simulink model "CF018A_GmRoadWhlInQlfr"  (R2013b)
settings: Solver=FixedStepDiscrete  SolverMode=SingleTasking  StartTime=0.0  StopTime=1  FixedStep=0.002  RelTol=1e-3
values from neighbouring files (symbols this model uses):
  DELTAPLSROLLOVR_CNT_S16 = DataDict.Constant    [CF018A_GmRoadWhlInQlfr_DataDict.m]
  DELTATISTAMPCNTROLLOVR_CNT_S32 = DataDict.Constant    [CF018A_GmRoadWhlInQlfr_DataDict.m]
  GmRoadWhlInQlfrMaxAllwblFrq = DataDict.Calibration    [CF018A_GmRoadWhlInQlfr_DataDict.m]
  GmRoadWhlInQlfrMaxFrqChg = DataDict.Calibration    [CF018A_GmRoadWhlInQlfr_DataDict.m]
  LEFRQCHGOUTOFRNG_CNT_U08 = DataDict.Constant    [CF018A_GmRoadWhlInQlfr_DataDict.m]
  LEFRQOUTOFRNG_CNT_U08 = DataDict.Constant    [CF018A_GmRoadWhlInQlfr_DataDict.m]
  NODEBSTEP_CNT_U16 = DataDict.Constant    [CF018A_GmRoadWhlInQlfr_DataDict.m]
  PARKDURN_CNT_F32 = DataDict.Constant    [CF018A_GmRoadWhlInQlfr_DataDict.m]
  PREVRAWWHLFRQMIN_HZ_F32 = DataDict.Constant    [CF018A_GmRoadWhlInQlfr_DataDict.m]
  RIFRQCHGOUTOFRNG_CNT_U08 = DataDict.Constant    [CF018A_GmRoadWhlInQlfr_DataDict.m]
  RIFRQOUTOFRNG_CNT_U08 = DataDict.Constant    [CF018A_GmRoadWhlInQlfr_DataDict.m]
  RoadWhlFrqInCalcOutOfRng = DataDict.NTC    [CF018A_GmRoadWhlInQlfr_DataDict.m]
  SECTO100MICROSECCNVN_CNT_F32 = DataDict.Constant    [CF018A_GmRoadWhlInQlfr_DataDict.m]
  WHLFRQMIN_HZ_F32 = DataDict.Constant    [CF018A_GmRoadWhlInQlfr_DataDict.m]
undefined symbols (not defined in the file or in its folder): NtcSts1
libraries: simulink x5, NxtrAbslt x2, NxtrLim x2
(part 3 of 5)

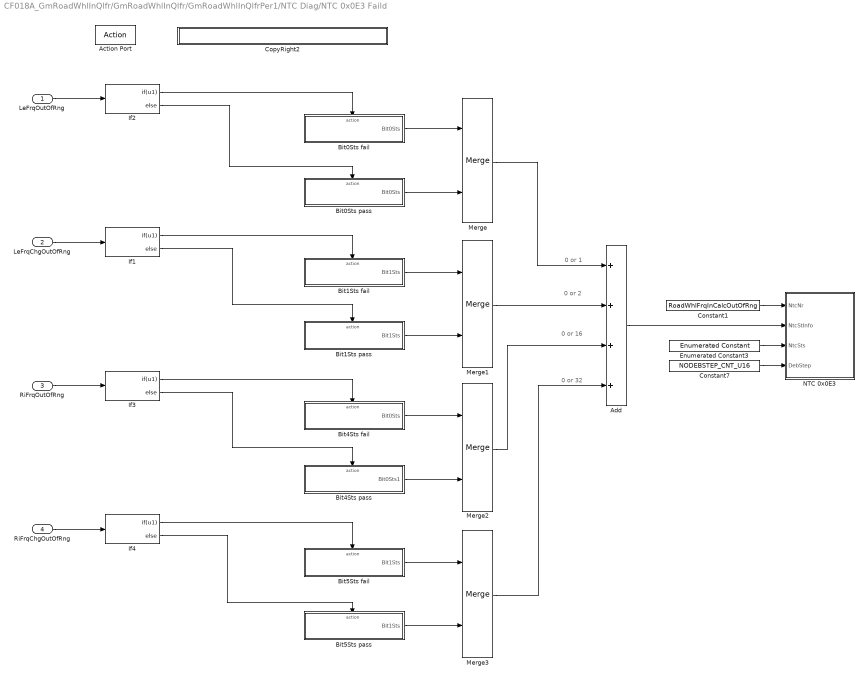
== system CF018A_GmRoadWhlInQlfr/GmRoadWhlInQlfr/GmRoadWhlInQlfrPer1/NTC Diag/NTC 0x0E3 Faild ==
  note: 0 or 32
  note: 0 or 16
  note: 0 or 2
  note: 0 or 1
  LeFrqOutOfRng : Inport  RequirementInfo="{'linktype_rmi_doors' '0000c6e7 (/GM T1XX/SubSystem Specifications/Customer Functions/CF018A GM Road Wheel Input Qualifier)' '#217' 'true' 'REQ:  217' '' } %GIDa_195ab2bc_dfff_4d6d_a0a2_4361903f55fa"
  LeFrqChgOutOfRng : Inport  RequirementInfo="{'linktype_rmi_doors' '0000c6e7 (/GM T1XX/SubSystem Specifications/Customer Functions/CF018A GM Road Wheel Input Qualifier)' '#219' 'true' 'REQ:  219' '' } %GIDa_52460b67_ef53_458f_9626_54e9bbcdf812"  Port=2
  RiFrqOutOfRng : Inport  RequirementInfo="{'linktype_rmi_doors' '0000c6e7 (/GM T1XX/SubSystem Specifications/Customer Functions/CF018A GM Road Wheel Input Qualifier)' '#220' 'true' 'REQ:  220' '' } %GIDa_71d41fd8_1e3e_427a_97ad_955d8ac34ef3"  Port=3
  RiFrqChgOutOfRng : Inport  RequirementInfo="{'linktype_rmi_doors' '0000c6e7 (/GM T1XX/SubSystem Specifications/Customer Functions/CF018A GM Road Wheel Input Qualifier)' '#221' 'true' 'REQ:  221' '' } %GIDa_232d1f07_579d_47ef_90f3_e50f36280ea6"  Port=4
  Action Port : ActionPort  ActionType=then
  Add : Sum  Inputs=++++
  Bit0Sts fail : Subsystem  RequirementInfo="{'linktype_rmi_doors' '0000c6e7 (/GM T1XX/SubSystem Specifications/Customer Functions/CF018A GM Road Wheel Input Qualifier)' '#217' 'true' 'REQ:  217' '' } %GIDa_14e418d7_b229_4493_b7eb_676a8f1cb482"  TreatAsAtomicUnit=on
  Bit0Sts pass : Subsystem  RequirementInfo="{'linktype_rmi_doors' '0000c6e7 (/GM T1XX/SubSystem Specifications/Customer Functions/CF018A GM Road Wheel Input Qualifier)' '#217' 'true' 'REQ:  217' '' } %GIDa_4b309baa_eb20_4fda_8a66_476882cf3a3c"  TreatAsAtomicUnit=on
  Bit1Sts fail : Subsystem  RequirementInfo="{'linktype_rmi_doors' '0000c6e7 (/GM T1XX/SubSystem Specifications/Customer Functions/CF018A GM Road Wheel Input Qualifier)' '#219' 'true' 'REQ:  219' '' } %GIDa_385de269_cf1d_4f17_ae75_b6c4c0e42b90"  TreatAsAtomicUnit=on
  Bit1Sts pass : Subsystem  RequirementInfo="{'linktype_rmi_doors' '0000c6e7 (/GM T1XX/SubSystem Specifications/Customer Functions/CF018A GM Road Wheel Input Qualifier)' '#219' 'true' 'REQ:  219' '' } %GIDa_8ec329c6_93d5_43d4_8a4f_e98046b859d6"  TreatAsAtomicUnit=on
  Bit4Sts fail : Subsystem  RequirementInfo="{'linktype_rmi_doors' '0000c6e7 (/GM T1XX/SubSystem Specifications/Customer Functions/CF018A GM Road Wheel Input Qualifier)' '#220' 'true' 'REQ:  220' '' } %GIDa_b3b904ac_bc0c_48f5_a89a_5cd3c3707194"  TreatAsAtomicUnit=on
  Bit4Sts pass : Subsystem  RequirementInfo="{'linktype_rmi_doors' '0000c6e7 (/GM T1XX/SubSystem Specifications/Customer Functions/CF018A GM Road Wheel Input Qualifier)' '#220' 'true' 'REQ:  220' '' } %GIDa_da90ecd1_a52b_401f_93fe_b339ee453102"  TreatAsAtomicUnit=on
  Bit5Sts fail : Subsystem  RequirementInfo="{'linktype_rmi_doors' '0000c6e7 (/GM T1XX/SubSystem Specifications/Customer Functions/CF018A GM Road Wheel Input Qualifier)' '#221' 'true' 'REQ:  221' '' } %GIDa_36f13dc0_335a_4247_a7fa_e2ce04f25d73"  TreatAsAtomicUnit=on
  Bit5Sts pass : Subsystem  RequirementInfo="{'linktype_rmi_doors' '0000c6e7 (/GM T1XX/SubSystem Specifications/Customer Functions/CF018A GM Road Wheel Input Qualifier)' '#221' 'true' 'REQ:  221' '' } %GIDa_8dbc0c8d_e7dc_445e_adc9_a51dc08e9455"  TreatAsAtomicUnit=on
  Constant1 : Constant  Value=RoadWhlFrqInCalcOutOfRng
  Constant7 : Constant  Value=NODEBSTEP_CNT_U16
  CopyRight2 : Subsystem  Description=|  mask(Copyright Information){none=on}
      | Copyright info block.                                               
      |                                                                     
      | Place copyright information at the top of every subsystem in design.
      mask prompts: none "No parameters"
      mask help: Place copyright information at the top of every subsystem in design.
      mask Display:
      | NxtrConf = 'Nexteer Confidential';
      | 
      | sys = bdroot; %handle for the current model ("system")
      | first = get_param(sys,'Created');
      | if(isempty(first))
      |     first = datestr(now,'yyyy');
      | else
      |     first = first(end-3:end);  %year is last four digits
      | end
      | 
      | last = get_param(sys,'LastModifiedDate');
      | if isempty(last)
      |     last = datestr(now,'yyyy');
      | else
      |     last = last(end-3:end);
      | end
      | 
      | if strcmp(first,last)
      |     fprintf('%s -- Copyright %s Nexteer',NxtrConf,first)
      | else
      |     fprintf('%s -- %s%s- %s Nexteer',NxtrConf,char(169),first,last)
      | end
  Enumerated Constant3 : simulink/Sources/Enumerated Constant  OutDataTypeStr=Enum: NtcSts1  Value=NtcSts1.NTCSTS_FAILD  SampleTime=inf
  If1 : If  RequirementInfo="{'linktype_rmi_doors' '0000c6e7 (/GM T1XX/SubSystem Specifications/Customer Functions/CF018A GM Road Wheel Input Qualifier)' '#219' 'true' 'REQ:  219' '' } %GIDa_aff6807a_1779_44a1_bb5d_bde3c1762c20"  IfExpression=u1
  If2 : If  RequirementInfo="{'linktype_rmi_doors' '0000c6e7 (/GM T1XX/SubSystem Specifications/Customer Functions/CF018A GM Road Wheel Input Qualifier)' '#217' 'true' 'REQ:  217' '' } %GIDa_a1263e25_a3bc_4e7a_be4f_bbb224f699c2"  IfExpression=u1
  If3 : If  RequirementInfo="{'linktype_rmi_doors' '0000c6e7 (/GM T1XX/SubSystem Specifications/Customer Functions/CF018A GM Road Wheel Input Qualifier)' '#220' 'true' 'REQ:  220' '' } %GIDa_0718b7b5_3f2c_43be_9873_dfe0614914d9"  IfExpression=u1
  If4 : If  RequirementInfo="{'linktype_rmi_doors' '0000c6e7 (/GM T1XX/SubSystem Specifications/Customer Functions/CF018A GM Road Wheel Input Qualifier)' '#221' 'true' 'REQ:  221' '' } %GIDa_596e93e5_c856_4c8d_b061_564bb26e16d1"  IfExpression=u1
  Merge : Merge  RequirementInfo="{'linktype_rmi_doors' '0000c6e7 (/GM T1XX/SubSystem Specifications/Customer Functions/CF018A GM Road Wheel Input Qualifier)' '#217' 'true' 'REQ:  217' '' } %GIDa_ff64cedf_763d_4ec6_811f_3d7fe7e08dc9"
  Merge1 : Merge  RequirementInfo="{'linktype_rmi_doors' '0000c6e7 (/GM T1XX/SubSystem Specifications/Customer Functions/CF018A GM Road Wheel Input Qualifier)' '#219' 'true' 'REQ:  219' '' } %GIDa_d687efa6_6282_443c_95ea_f8a69d949498"
  Merge2 : Merge  RequirementInfo="{'linktype_rmi_doors' '0000c6e7 (/GM T1XX/SubSystem Specifications/Customer Functions/CF018A GM Road Wheel Input Qualifier)' '#220' 'true' 'REQ:  220' '' } %GIDa_a420e449_a616_43ba_b126_66db9afefef1"
  Merge3 : Merge  RequirementInfo="{'linktype_rmi_doors' '0000c6e7 (/GM T1XX/SubSystem Specifications/Customer Functions/CF018A GM Road Wheel Input Qualifier)' '#221' 'true' 'REQ:  221' '' } %GIDa_6aea80f1_e3e4_4567_b723_2621865e42b7"
  NTC 0x0E3 : Subsystem  mask(SetNTC){}
      mask help: SetNTC library block
  wires:
  LeFrqOutOfRng/1 -> If2/1
  LeFrqChgOutOfRng/1 -> If1/1
  RiFrqOutOfRng/1 -> If3/1
  RiFrqChgOutOfRng/1 -> If4/1
  If2/1 -> Bit0Sts fail/Action
  If2/2 -> Bit0Sts pass/Action
  If1/1 -> Bit1Sts fail/Action
  If1/2 -> Bit1Sts pass/Action
  If3/1 -> Bit4Sts fail/Action
  If3/2 -> Bit4Sts pass/Action
  If4/1 -> Bit5Sts fail/Action
  If4/2 -> Bit5Sts pass/Action
  Bit0Sts fail/1(Bit0Sts) -> Merge/1
  Bit0Sts pass/1(Bit0Sts) -> Merge/2
  Bit1Sts fail/1(Bit1Sts) -> Merge1/1
  Bit1Sts pass/1(Bit1Sts) -> Merge1/2
  Bit4Sts fail/1(Bit0Sts) -> Merge2/1
  Bit4Sts pass/1(Bit0Sts1) -> Merge2/2
  Bit5Sts fail/1(Bit1Sts) -> Merge3/1
  Bit5Sts pass/1(Bit1Sts) -> Merge3/2
  Merge/1 -> Add/1
  Merge1/1 -> Add/2
  Merge2/1 -> Add/3
  Merge3/1 -> Add/4
  Enumerated Constant3/1 -> NTC 0x0E3/3(NtcSts)
  Constant7/1 -> NTC 0x0E3/4(DebStep)
  Add/1 -> NTC 0x0E3/2(NtcStInfo)
  Constant1/1 -> NTC 0x0E3/1(NtcNr)

== system CF018A_GmRoadWhlInQlfr/GmRoadWhlInQlfr/GmRoadWhlInQlfrPer1/NTC Diag/NTC 0x0E3 Passd ==
  NtcNr : Inport
  NtcStInfo : Inport  Port=2
  NtcSts : Inport  Port=3
  DebStep : Inport  Port=4
  CallDiagMgr : ActionPort  ActionType=else
  SetNtcSts : Subsystem  RequirementInfo={} %GIDa_11b0bea6_d358_4d89_9e51_342e19f776d7  TreatAsAtomicUnit=on
      settings: RTWSystemCode=Inline
  wires:
  NtcStInfo/1 -> SetNtcSts/2(NtcStInfo)
  DebStep/1 -> SetNtcSts/4(DebStep)
  NtcSts/1 -> SetNtcSts/3(NtcSts)
  NtcNr/1 -> SetNtcSts/1(NtcNr)  "NtcNr"

== system CF018A_GmRoadWhlInQlfr/GmRoadWhlInQlfr/GmRoadWhlInQlfrPer1/Set Min Le whl Frq and false /CopyRight2 ==

== system CF018A_GmRoadWhlInQlfr/GmRoadWhlInQlfr/GmRoadWhlInQlfrPer1/Set Min Ri whl Frq and false /CopyRight2 ==

== system CF018A_GmRoadWhlInQlfr/GmRoadWhlInQlfr/GmRoadWhlInQlfrInit1/NTC 0x0E3 Passd/SetNtcSts/CopyRight2 ==

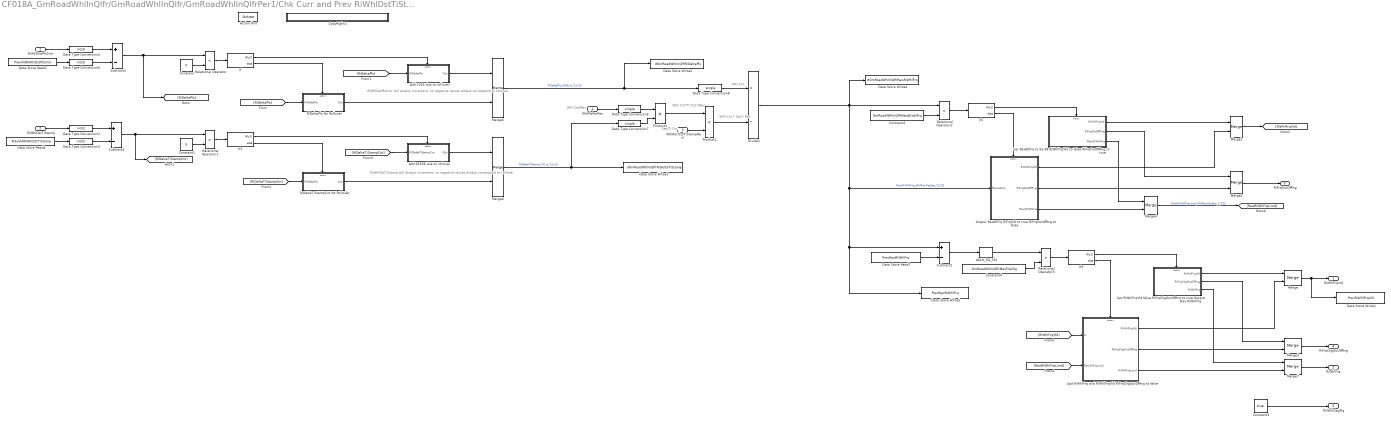
== system CF018A_GmRoadWhlInQlfr/GmRoadWhlInQlfr/GmRoadWhlInQlfrPer1/Chk Curr and Prev RiWhlDstTiStamp/Calc RiWhlFrq and RiWhlFrqVld /Calc RiWhlFrq and RiWhlFrqVld  ==
  note: RiWhlDstPlsCntr will always increment, so negative values always correspond to rollover
  note: RiWhlDstTiStamp will always increment, so negative values always correspond to rollover
  note: Whl Cnt/Rev
  note: Whl Cnt
  note: (Whl Cnt * Sec)/ Rev
  note: (Whl Cnt*Ti Cnt)/Rev
  note: Sec/Ti Cnt
  RiWhlDstPlsCntr : Inport  RequirementInfo="{'linktype_rmi_doors' '0000c6e7 (/GM T1XX/SubSystem Specifications/Customer Functions/CF018A GM Road Wheel Input Qualifier)' '#193' 'true' 'REQ:  193' '' } %GIDa_3e8ab2e0_17e6_46c6_9b5a_a415c584676f"
  RiWhlDstTiStamp : Inport  RequirementInfo="{'linktype_rmi_doors' '0000c6e7 (/GM T1XX/SubSystem Specifications/Customer Functions/CF018A GM Road Wheel Input Qualifier)' '#193' 'true' 'REQ:  193' '' } %GIDa_5cc4ad43_c4fb_48e7_9d1a_97e50fd9bb1d"  Port=2
  WhlRotlStsTiStampResl : Inport  RequirementInfo="{'linktype_rmi_doors' '0000c6e7 (/GM T1XX/SubSystem Specifications/Customer Functions/CF018A GM Road Wheel Input Qualifier)' '#193' 'true' 'REQ:  193' '' } %GIDa_18c1bb4c_4f3d_4131_89e1_1f0c775e5c47"  Port=3
  WhlPlsPerRev : Inport  RequirementInfo="{'linktype_rmi_doors' '0000c6e7 (/GM T1XX/SubSystem Specifications/Customer Functions/CF018A GM Road Wheel Input Qualifier)' '#193' 'true' 'REQ:  193' '' } %GIDa_22c598b2_0977_47f8_84d1_6d93f9add662"  Port=4
  Action Port : ActionPort  ActionType=then
  Abslt_f32_f32 : NxtrAbslt/Abslt_f32_f32  RequirementInfo="{'linktype_rmi_doors' '0000c6e7 (/GM T1XX/SubSystem Specifications/Customer Functions/CF018A GM Road Wheel Input Qualifier)' '#195' 'true' 'REQ:  195' '' } %GIDa_b87ef623_fea8_40fc_be2f_01a19a2481d3"  SFunctionSpec=single y1 = Abslt_f32_f32(single u1)
      settings: AttributesFormatString=%<Name>
  Add 1024 due to rollover : Subsystem  RequirementInfo="{'linktype_rmi_doors' '0000c6e7 (/GM T1XX/SubSystem Specifications/Customer Functions/CF018A GM Road Wheel Input Qualifier)' '#193' 'true' 'REQ:  193' '' } %GIDa_bbe013d7_37c0_4606_a70f_3e626e7cf5b9"  TreatAsAtomicUnit=on
  Add 65536 due to rollover : Subsystem  RequirementInfo="{'linktype_rmi_doors' '0000c6e7 (/GM T1XX/SubSystem Specifications/Customer Functions/CF018A GM Road Wheel Input Qualifier)' '#193' 'true' 'REQ:  193' '' } %GIDa_8f11591a_3e36_4330_89d4_3e165bb1c8e4"  TreatAsAtomicUnit=on
  Constant : Constant  RequirementInfo="{'linktype_rmi_doors' '0000c6e7 (/GM T1XX/SubSystem Specifications/Customer Functions/CF018A GM Road Wheel Input Qualifier)' '#193' 'true' 'REQ:  193' '' } %GIDa_b5ba1cba_4aae_479b_830a_1e93dfe9f490"  Value=0  OutDataTypeStr=int16
  Constant1 : Constant  RequirementInfo="{'linktype_rmi_doors' '0000c6e7 (/GM T1XX/SubSystem Specifications/Customer Functions/CF018A GM Road Wheel Input Qualifier)' '#193' 'true' 'REQ:  193' '' } %GIDa_e84f4047_7d95_4eef_aeae_45f6caa05096"  Value=0
  Constant2 : Constant  RequirementInfo="{'linktype_rmi_doors' '0000c6e7 (/GM T1XX/SubSystem Specifications/Customer Functions/CF018A GM Road Wheel Input Qualifier)' '#218' 'true' 'REQ:  218' '' ; 'linktype_rmi_doors' '0000c6e7 (/GM T1XX/SubSystem Specifications/Customer Functions/CF018A GM Road Wheel Input Qualifier)' '#194' 'true' 'REQ:  194' '' } %GIDa_09ac7b7c_57cd_4577_93bc_6054e9bf264a"  Value=GmRoadWhlInQlfrMaxAllwblFrq  OutDataTypeStr=single
  Constant3 : Constant  Value=true  OutDataTypeStr=boolean
      settings: AttributesFormatString=%<OutDataTypeStr>
  Constant4 : Constant  RequirementInfo="{'linktype_rmi_doors' '0000c6e7 (/GM T1XX/SubSystem Specifications/Customer Functions/CF018A GM Road Wheel Input Qualifier)' '#195' 'true' 'REQ:  195' '' } %GIDa_37fdba2b_4f11_40e7_bf62_90e20809034e"  Value=GmRoadWhlInQlfrMaxFrqChg
  CopyRight2 : Subsystem  Description=|  mask(Copyright Information){none=on}
      | Copyright info block.                                               
      |                                                                     
      | Place copyright information at the top of every subsystem in design.
      mask prompts: none "No parameters"
      mask help: Place copyright information at the top of every subsystem in design.
      mask Display:
      | NxtrConf = 'Nexteer Confidential';
      | 
      | sys = bdroot; %handle for the current model ("system")
      | first = get_param(sys,'Created');
      | if(isempty(first))
      |     first = datestr(now,'yyyy');
      | else
      |     first = first(end-3:end);  %year is last four digits
      | end
      | 
      | last = get_param(sys,'LastModifiedDate');
      | if isempty(last)
      |     last = datestr(now,'yyyy');
      | else
      |     last = last(end-3:end);
      | end
      | 
      | if strcmp(first,last)
      |     fprintf('%s -- Copyright %s Nexteer',NxtrConf,first)
      | else
      |     fprintf('%s -- %s%s- %s Nexteer',NxtrConf,char(169),first,last)
      | end
  Data Store Read1 : DataStoreRead  RequirementInfo="{'linktype_rmi_doors' '0000c6e7 (/GM T1XX/SubSystem Specifications/Customer Functions/CF018A GM Road Wheel Input Qualifier)' '#193' 'true' 'REQ:  193' '' } %GIDa_797000f7_ce4b_4c5c_a521_331a1c1a42ab"  DataStoreName=PrevVldRiWhlDstPlsCntr
  Data Store Read4 : DataStoreRead  RequirementInfo="{'linktype_rmi_doors' '0000c6e7 (/GM T1XX/SubSystem Specifications/Customer Functions/CF018A GM Road Wheel Input Qualifier)' '#193' 'true' 'REQ:  193' '' } %GIDa_1fb5ca86_d0de_4e3c_9635_5292953ee6b0"  DataStoreName=PrevVldRiWhlDstTiStamp
  Data Store Read7 : DataStoreRead  RequirementInfo="{'linktype_rmi_doors' '0000c6e7 (/GM T1XX/SubSystem Specifications/Customer Functions/CF018A GM Road Wheel Input Qualifier)' '#195' 'true' 'REQ:  195' '' } %GIDa_812f6d58_6b1c_477d_90ab_6c8a1329252d"  Priority=0  DataStoreName=PrevRawRiWhlFrq
      settings: AttributesFormatString=%<Priority>
  Data Store Write1 : DataStoreWrite  RequirementInfo="{'linktype_rmi_doors' '0000c6e7 (/GM T1XX/SubSystem Specifications/Customer Functions/CF018A GM Road Wheel Input Qualifier)' '#195' 'true' 'REQ:  195' '' } %GIDa_9705072b_21fb_4b74_9645_80877c8d3669"  DataStoreName=PrevRiWhlFrqVld
      settings: AttributesFormatString=%<Priority>
  Data Store Write2 : DataStoreWrite  RequirementInfo="{'linktype_rmi_doors' '0000c6e7 (/GM T1XX/SubSystem Specifications/Customer Functions/CF018A GM Road Wheel Input Qualifier)' '#193' 'true' 'REQ:  193' '' } %GIDa_07565cfc_dc92_4065_822c_72345d7434ef"  DataStoreName=dGmRoadWhlInQlfrRiDeltaPls
  Data Store Write3 : DataStoreWrite  RequirementInfo="{'linktype_rmi_doors' '0000c6e7 (/GM T1XX/SubSystem Specifications/Customer Functions/CF018A GM Road Wheel Input Qualifier)' '#193' 'true' 'REQ:  193' '' } %GIDa_122dcde5_ac2e_4abf_941f_12224557870d"  DataStoreName=dGmRoadWhlInQlfrRiDeltaTiStamp
  Data Store Write4 : DataStoreWrite  RequirementInfo="{'linktype_rmi_doors' '0000c6e7 (/GM T1XX/SubSystem Specifications/Customer Functions/CF018A GM Road Wheel Input Qualifier)' '#194' 'true' 'REQ:  194' '' } %GIDa_96150977_36bd_4448_a7f7_af42a0980b08"  DataStoreName=dGmRoadWhlInQlfrRawRiWhlFrq
  Data Store Write5 : DataStoreWrite  RequirementInfo="{'linktype_rmi_doors' '0000c6e7 (/GM T1XX/SubSystem Specifications/Customer Functions/CF018A GM Road Wheel Input Qualifier)' '#195' 'true' 'REQ:  195' '' } %GIDa_a6dec644_92a4_4cb8_bf15_67a29e16d7d6"  Priority=1  DataStoreName=PrevRawRiWhlFrq
      settings: AttributesFormatString=%<Priority>
  Data Type Conversion2 : DataTypeConversion  OutDataTypeStr=int32
  Data Type Conversion3 : DataTypeConversion  OutDataTypeStr=int32
  Data Type Conversion4 : DataTypeConversion  OutDataTypeStr=int16
  Data Type Conversion5 : DataTypeConversion  RequirementInfo="{'linktype_rmi_doors' '0000c6e7 (/GM T1XX/SubSystem Specifications/Customer Functions/CF018A GM Road Wheel Input Qualifier)' '#170' 'true' 'REQ:  170' '' } %GIDa_e7ae9d6c_fed1_4580_98f9_e45e50ba6ceb"  OutDataTypeStr=single
  Data Type Conversion6 : DataTypeConversion  OutDataTypeStr=int16
  Data Type Conversion7 : DataTypeConversion  RequirementInfo="{'linktype_rmi_doors' '0000c6e7 (/GM T1XX/SubSystem Specifications/Customer Functions/CF018A GM Road Wheel Input Qualifier)' '#170' 'true' 'REQ:  170' '' } %GIDa_0818f86b_9f57_42d4_8b68_d1a575d3be0e"  OutDataTypeStr=single
  Data Type Conversion8 : DataTypeConversion  RequirementInfo="{'linktype_rmi_doors' '0000c6e7 (/GM T1XX/SubSystem Specifications/Customer Functions/CF018A GM Road Wheel Input Qualifier)' '#170' 'true' 'REQ:  170' '' } %GIDa_2241e601_1dcd_401c_a59f_e8ade4dc7a60"  OutDataTypeStr=single
  Divide1 : Product  RequirementInfo="{'linktype_rmi_doors' '0000c6e7 (/GM T1XX/SubSystem Specifications/Customer Functions/CF018A GM Road Wheel Input Qualifier)' '#193' 'true' 'REQ:  193' '' } %GIDa_472150d3_7fbc_4109_9c55_3e48dd5b6845"  Inputs=*/
      settings: AttributesFormatString=%<Priority>
  If : If  RequirementInfo="{'linktype_rmi_doors' '0000c6e7 (/GM T1XX/SubSystem Specifications/Customer Functions/CF018A GM Road Wheel Input Qualifier)' '#193' 'true' 'REQ:  193' '' } %GIDa_1801537b_4966_4c64_9561_2cee048af28c"  IfExpression=u1
  If1 : If  RequirementInfo="{'linktype_rmi_doors' '0000c6e7 (/GM T1XX/SubSystem Specifications/Customer Functions/CF018A GM Road Wheel Input Qualifier)' '#193' 'true' 'REQ:  193' '' } %GIDa_42eb8486_ab3d_4fa1_9a03_938fcd0c4e30"  IfExpression=u1
  If2 : If  RequirementInfo="{'linktype_rmi_doors' '0000c6e7 (/GM T1XX/SubSystem Specifications/Customer Functions/CF018A GM Road Wheel Input Qualifier)' '#194' 'true' 'REQ:  194' '' } %GIDa_a57bee02_ce77_48d2_88cd_7c4ae3532c41"  IfExpression=u1
  If3 : If  RequirementInfo="{'linktype_rmi_doors' '0000c6e7 (/GM T1XX/SubSystem Specifications/Customer Functions/CF018A GM Road Wheel Input Qualifier)' '#195' 'true' 'REQ:  195' '' } %GIDa_08ef704c_fbdc_4660_8593_39b9eaa85229"  IfExpression=u1
  Merge : Merge  RequirementInfo="{'linktype_rmi_doors' '0000c6e7 (/GM T1XX/SubSystem Specifications/Customer Functions/CF018A GM Road Wheel Input Qualifier)' '#195' 'true' 'REQ:  195' '' } %GIDa_e2ef6487_5991_4c3a_a631_564a79c2fe86"
  Merge1 : Merge  RequirementInfo="{'linktype_rmi_doors' '0000c6e7 (/GM T1XX/SubSystem Specifications/Customer Functions/CF018A GM Road Wheel Input Qualifier)' '#194' 'true' 'REQ:  194' '' } %GIDa_e41c48f7_6ec3_4d13_b960_474c261889e6"
  Merge2 : Merge  RequirementInfo="{'linktype_rmi_doors' '0000c6e7 (/GM T1XX/SubSystem Specifications/Customer Functions/CF018A GM Road Wheel Input Qualifier)' '#194' 'true' 'REQ:  194' '' } %GIDa_c24260f6_a763_412a_9b57_2a3beb947fdf"
  Merge3 : Merge  RequirementInfo="{'linktype_rmi_doors' '0000c6e7 (/GM T1XX/SubSystem Specifications/Customer Functions/CF018A GM Road Wheel Input Qualifier)' '#195' 'true' 'REQ:  195' '' } %GIDa_bb8419c7_3cbc_425c_86e3_43eeea52c995"
  Merge4 : Merge  RequirementInfo="{'linktype_rmi_doors' '0000c6e7 (/GM T1XX/SubSystem Specifications/Customer Functions/CF018A GM Road Wheel Input Qualifier)' '#194' 'true' 'REQ:  194' '' } %GIDa_6a451dcf_a05f_4d42_aef8_a73a6e5c3b13"
  Merge5 : Merge  RequirementInfo="{'linktype_rmi_doors' '0000c6e7 (/GM T1XX/SubSystem Specifications/Customer Functions/CF018A GM Road Wheel Input Qualifier)' '#193' 'true' 'REQ:  193' '' } %GIDa_ccfc636f_400d_44cf_b737_482d710de06b"
  Merge6 : Merge  RequirementInfo="{'linktype_rmi_doors' '0000c6e7 (/GM T1XX/SubSystem Specifications/Customer Functions/CF018A GM Road Wheel Input Qualifier)' '#193' 'true' 'REQ:  193' '' } %GIDa_c5d7f19d_bf6a_4178_8121_009387576404"
  Merge7 : Merge  RequirementInfo="{'linktype_rmi_doors' '0000c6e7 (/GM T1XX/SubSystem Specifications/Customer Functions/CF018A GM Road Wheel Input Qualifier)' '#195' 'true' 'REQ:  195' '' } %GIDa_daec4de5_ff8c_4e15_b55d_7ce836035153"
  Output RawRiFrq RiFrqVld to true RiFrqOutOfRng to false : Subsystem  RequirementInfo="{'linktype_rmi_doors' '0000c6e7 (/GM T1XX/SubSystem Specifications/Customer Functions/CF018A GM Road Wheel Input Qualifier)' '#194' 'true' 'REQ:  194' '' } %GIDa_593ffa87_d2e3_4775_b9e7_b2900ff43455"  TreatAsAtomicUnit=on
  Product1 : Product  RequirementInfo="{'linktype_rmi_doors' '0000c6e7 (/GM T1XX/SubSystem Specifications/Customer Functions/CF018A GM Road Wheel Input Qualifier)' '#193' 'true' 'REQ:  193' '' } %GIDa_27b08f6a_668b_431d_8df5_c3d021ac0bd2"
  Product2 : Product  RequirementInfo="{'linktype_rmi_doors' '0000c6e7 (/GM T1XX/SubSystem Specifications/Customer Functions/CF018A GM Road Wheel Input Qualifier)' '#193' 'true' 'REQ:  193' '' } %GIDa_3d707914_3235_42a9_aa8d_b9d485065294"
  Relational Operator : RelationalOperator  RequirementInfo="{'linktype_rmi_doors' '0000c6e7 (/GM T1XX/SubSystem Specifications/Customer Functions/CF018A GM Road Wheel Input Qualifier)' '#193' 'true' 'REQ:  193' '' } %GIDa_49ec36b8_3bec_4187_b4ff_6880b6263c69"  Operator=<  OutDataTypeStr=boolean
  Relational Operator1 : RelationalOperator  RequirementInfo="{'linktype_rmi_doors' '0000c6e7 (/GM T1XX/SubSystem Specifications/Customer Functions/CF018A GM Road Wheel Input Qualifier)' '#193' 'true' 'REQ:  193' '' } %GIDa_a83cc7e3_4e80_4fa3_b12c_790291f5afb3"  Operator=<  OutDataTypeStr=boolean
  Relational Operator2 : RelationalOperator  RequirementInfo="{'linktype_rmi_doors' '0000c6e7 (/GM T1XX/SubSystem Specifications/Customer Functions/CF018A GM Road Wheel Input Qualifier)' '#194' 'true' 'REQ:  194' '' } %GIDa_e7396e0f_cc94_481e_9045_3adb35a10baf"  Operator=>  OutDataTypeStr=boolean
  Relational Operator3 : RelationalOperator  RequirementInfo="{'linktype_rmi_doors' '0000c6e7 (/GM T1XX/SubSystem Specifications/Customer Functions/CF018A GM Road Wheel Input Qualifier)' '#195' 'true' 'REQ:  195' '' } %GIDa_a6de90ed_f03a_4890_9d62_a519069a7561"  Operator=>  OutDataTypeStr=boolean
  RiDeltaPls No Rollover : Subsystem  RequirementInfo="{'linktype_rmi_doors' '0000c6e7 (/GM T1XX/SubSystem Specifications/Customer Functions/CF018A GM Road Wheel Input Qualifier)' '#193' 'true' 'REQ:  193' '' } %GIDa_93c1926d_7fde_48a6_a163_aa619db4a291"  TreatAsAtomicUnit=on
  RiDeltaTiStampCnt No Rollover : Subsystem  RequirementInfo="{'linktype_rmi_doors' '0000c6e7 (/GM T1XX/SubSystem Specifications/Customer Functions/CF018A GM Road Wheel Input Qualifier)' '#193' 'true' 'REQ:  193' '' } %GIDa_f8733acd_867e_44dc_b8ac_27e7f0fa101f"  TreatAsAtomicUnit=on
  Set RawRiFrq to 55.48 RiWhlFrqVld to false RiFrqOutOfRng to true : Subsystem  RequirementInfo="{'linktype_rmi_doors' '0000c6e7 (/GM T1XX/SubSystem Specifications/Customer Functions/CF018A GM Road Wheel Input Qualifier)' '#194' 'true' 'REQ:  194' '' } %GIDa_703e1cf8_4d27_4088_a620_405ef56a5e54"  TreatAsAtomicUnit=on
  Set RiWhlFrqVld false RiFrqChgOutOfRng to true Output Prev RiWhlFrq : Subsystem  RequirementInfo="{'linktype_rmi_doors' '0000c6e7 (/GM T1XX/SubSystem Specifications/Customer Functions/CF018A GM Road Wheel Input Qualifier)' '#195' 'true' 'REQ:  195' '' } %GIDa_9eb7ff64_f26e_4233_94fd_148683f59f0b"  TreatAsAtomicUnit=on
  Subtract2 : Sum  RequirementInfo="{'linktype_rmi_doors' '0000c6e7 (/GM T1XX/SubSystem Specifications/Customer Functions/CF018A GM Road Wheel Input Qualifier)' '#195' 'true' 'REQ:  195' '' } %GIDa_1b5d7f40_849e_44f8_b97f_b5e560bb4383"  Inputs=+-
  Subtract3 : Sum  RequirementInfo="{'linktype_rmi_doors' '0000c6e7 (/GM T1XX/SubSystem Specifications/Customer Functions/CF018A GM Road Wheel Input Qualifier)' '#193' 'true' 'REQ:  193' '' } %GIDa_7b872e42_c67c_4581_bc3d_df00dad00f1b"  Inputs=+-  OutDataTypeStr=int16
      settings: AttributesFormatString=%<Priority>
  Subtract4 : Sum  RequirementInfo="{'linktype_rmi_doors' '0000c6e7 (/GM T1XX/SubSystem Specifications/Customer Functions/CF018A GM Road Wheel Input Qualifier)' '#193' 'true' 'REQ:  193' '' } %GIDa_bdde9b6a_5d40_4367_abef_413355ec8719"  Inputs=+-  OutDataTypeStr=int32
      settings: AttributesFormatString=%<Priority>
  Upd RiWhlFrq and RiWhlFrqVld RiFrqChgOutOfRng to false : Subsystem  RequirementInfo="{'linktype_rmi_doors' '0000c6e7 (/GM T1XX/SubSystem Specifications/Customer Functions/CF018A GM Road Wheel Input Qualifier)' '#195' 'true' 'REQ:  195' '' } %GIDa_b1fe3b64_95ed_4c02_b667_6eebcb10bf7c"  TreatAsAtomicUnit=on
  RiWhlFrqVld : Outport  RequirementInfo="{'linktype_rmi_doors' '0000c6e7 (/GM T1XX/SubSystem Specifications/Customer Functions/CF018A GM Road Wheel Input Qualifier)' '#195' 'true' 'REQ:  195' '' } %GIDa_75310a4e_8e01_451b_8bcc_d4d7b15e9f71"
  RiWhlFrq : Outport  RequirementInfo="{'linktype_rmi_doors' '0000c6e7 (/GM T1XX/SubSystem Specifications/Customer Functions/CF018A GM Road Wheel Input Qualifier)' '#195' 'true' 'REQ:  195' '' } %GIDa_9e2314b0_934c_42e1_9e05_95c79d3ea201"  Port=2
  RiFrqOutOfRng : Outport  RequirementInfo="{'linktype_rmi_doors' '0000c6e7 (/GM T1XX/SubSystem Specifications/Customer Functions/CF018A GM Road Wheel Input Qualifier)' '#194' 'true' 'REQ:  194' '' } %GIDa_09fb92da_568f_43be_b549_b57def9dc646"  Port=3
  RiFrqChgOutOfRng : Outport  RequirementInfo="{'linktype_rmi_doors' '0000c6e7 (/GM T1XX/SubSystem Specifications/Customer Functions/CF018A GM Road Wheel Input Qualifier)' '#195' 'true' 'REQ:  195' '' } %GIDa_3399ff42_7753_46fb_ac1c_8614d6e8bb21"  Port=4
  RiWhlDiagFlg : Outport  Port=5
  wires:
  Abslt_f32_f32/1 -> Relational Operator3/1
  Data Type Conversion8/1 -> Divide1/1
  If2/2 -> Output RawRiFrq RiFrqVld to true RiFrqOutOfRng to false/Action
  Merge/1 -> Data Store Write1/1, RiWhlFrqVld/1
  Set RiWhlFrqVld false RiFrqChgOutOfRng to true Output Prev RiWhlFrq/1(RiWhlFrqVld) -> Merge/1
  Upd RiWhlFrq and RiWhlFrqVld RiFrqChgOutOfRng to false/1(RiWhlFrqVld) -> Merge/2
  If3/2 -> Upd RiWhlFrq and RiWhlFrqVld RiFrqChgOutOfRng to false/Action
  If3/1 -> Set RiWhlFrqVld false RiFrqChgOutOfRng to true Output Prev RiWhlFrq/Action
  Subtract2/1 -> Abslt_f32_f32/1
  Relational Operator3/1 -> If3/1
  Constant4/1 -> Relational Operator3/2
  Data Store Read7/1 -> Subtract2/2
  Divide1/1 -> Data Store Write4/1, Subtract2/1, Data Store Write5/1, Output RawRiFrq RiFrqVld to true RiFrqOutOfRng to false/1(RawLeFrq), Relational Operator2/1  "RawRiWhlFrq_WhlRevPerSec_T_F32"
  If2/1 -> Set RawRiFrq to 55.48 RiWhlFrqVld to false RiFrqOutOfRng to true/Action
  Relational Operator2/1 -> If2/1
  Constant2/1 -> Relational Operator2/2
  Product2/1 -> Product1/1
  WhlRotlStsTiStampResl/1 -> Product1/2
  Constant1/1 -> Relational Operator1/2
  Relational Operator1/1 -> If1/1
  Data Store Read4/1 -> Data Type Conversion3/1
  If1/1 -> Add 65536 due to rollover/Action
  Constant/1 -> Relational Operator/2
  Relational Operator/1 -> If/1
  If/1 -> Add 1024 due to rollover/Action
  Product1/1 -> Divide1/2
  RiWhlDstPlsCntr/1 -> Data Type Conversion4/1
  Data Store Read1/1 -> Data Type Conversion6/1
  If/2 -> RiDeltaPls No Rollover/Action
  RiWhlDstTiStamp/1 -> Data Type Conversion2/1
  [RiDeltaPls] -> RiDeltaPls No Rollover/1(RiDeltaPls)
  [RiDeltaPls] -> Add 1024 due to rollover/1(RiDeltaPls)
  If1/2 -> RiDeltaTiStampCnt No Rollover/Action
  [RiDeltaTiStampCnt] -> RiDeltaTiStampCnt No Rollover/1(RiDeltaPls)
  [RiDeltaTiStampCnt] -> Add 65536 due to rollover/1(RiDeltaTiStampCnt)
  Subtract4/1 -> [RiDeltaTiStampCnt], Relational Operator1/1
  Subtract3/1 -> Relational Operator/1, [RiDeltaPls]
  Add 1024 due to rollover/1(Out) -> Merge5/1
  RiDeltaPls No Rollover/1(Out) -> Merge5/2
  Merge5/1 -> Data Type Conversion8/1, Data Store Write2/1  "RiDeltaPls_WhlCnt_T_U16"
  Add 65536 due to rollover/1(Out) -> Merge6/1
  RiDeltaTiStampCnt No Rollover/1(Out) -> Merge6/2
  Merge6/1 -> Data Type Conversion7/1, Data Store Write3/1  "RiDeltaTiStamp_TiCnt_T_U16"
  Set RawRiFrq to 55.48 RiWhlFrqVld to false RiFrqOutOfRng to true/1(RiWhlFrqVld) -> Merge1/1
  Output RawRiFrq RiFrqVld to true RiFrqOutOfRng to false/1(RiWhlFrqVld) -> Merge1/2
  Set RawRiFrq to 55.48 RiWhlFrqVld to false RiFrqOutOfRng to true/2(RiFrqOutOfRng) -> Merge2/1
  Output RawRiFrq RiFrqVld to true RiFrqOutOfRng to false/2(RiFrqOutOfRng) -> Merge2/2
  Set RawRiFrq to 55.48 RiWhlFrqVld to false RiFrqOutOfRng to true/3(RawRiWhlFrq) -> Merge4/1
  Output RawRiFrq RiFrqVld to true RiFrqOutOfRng to false/3(RawRiWhlFrq) -> Merge4/2
  Merge1/1 -> [RiWhlFrqVld]
  Merge2/1 -> RiFrqOutOfRng/1
  Merge4/1 -> [RawRiWhlFrqLimd]  "RawRiWhlFrqLimd_WhlRevPerSec_T_F32"
  [RiWhlFrqVld] -> Upd RiWhlFrq and RiWhlFrqVld RiFrqChgOutOfRng to false/1(In)
  [RawRiWhlFrqLimd] -> Upd RiWhlFrq and RiWhlFrqVld RiFrqChgOutOfRng to false/2(RawRiFrqLimd)
  Upd RiWhlFrq and RiWhlFrqVld RiFrqChgOutOfRng to false/2(RiFrqChgOutOfRng) -> Merge3/2
  Set RiWhlFrqVld false RiFrqChgOutOfRng to true Output Prev RiWhlFrq/2(RiFrqChgOutOfRng) -> Merge3/1
  Merge3/1 -> RiFrqChgOutOfRng/1
  Constant3/1 -> RiWhlDiagFlg/1
  Merge7/1 -> RiWhlFrq/1
  Set RiWhlFrqVld false RiFrqChgOutOfRng to true Output Prev RiWhlFrq/3(RiWhlFrq) -> Merge7/1
  Upd RiWhlFrq and RiWhlFrqVld RiFrqChgOutOfRng to false/3(RiWhlFrqLimd) -> Merge7/2
  Data Type Conversion2/1 -> Subtract4/1
  Data Type Conversion3/1 -> Subtract4/2
  WhlPlsPerRev/1 -> Data Type Conversion5/1
  Data Type Conversion7/1 -> Product2/2
  Data Type Conversion6/1 -> Subtract3/2
  Data Type Conversion4/1 -> Subtract3/1
  Data Type Conversion5/1 -> Product2/1

== system CF018A_GmRoadWhlInQlfr/GmRoadWhlInQlfr/GmRoadWhlInQlfrPer1/Chk Curr and Prev RiWhlDstTiStamp/Calc RiWhlFrq and RiWhlFrqVld /CopyRight2 ==

== system CF018A_GmRoadWhlInQlfr/GmRoadWhlInQlfr/GmRoadWhlInQlfrPer1/Chk Curr and Prev RiWhlDstTiStamp/Calc RiWhlFrq and RiWhlFrqVld /GetRefTmr100MicroSec32bit ==
  note: Created Aug 18, 2015
      | Modified Oct 21, 2015
      | Modified Oct 30, 2015
      | Kevin Derry
  note: GetRefTmr100MicroSec32bit
  note: Wrap-to-zero
  note: counts
  note: microseconds
  note: seconds
  note: 1 count = 100 uSec
  CopyRight2 : Subsystem  Description=|  mask(Copyright Information){none=on}
      | Copyright info block.                                               
      |                                                                     
      | Place copyright information at the top of every subsystem in design.
      mask prompts: none "No parameters"
      mask help: Place copyright information at the top of every subsystem in design.
      mask Display:
      | NxtrConf = 'Nexteer Confidential';
      | 
      | sys = bdroot; %handle for the current model ("system")
      | first = get_param(sys,'Created');
      | if(isempty(first))
      |     first = datestr(now,'yyyy');
      | else
      |     first = first(end-3:end);  %year is last four digits
      | end
      | 
      | last = get_param(sys,'LastModifiedDate');
      | if isempty(last)
      |     last = datestr(now,'yyyy');
      | else
      |     last = last(end-3:end);
      | end
      | 
      | if strcmp(first,last)
      |     fprintf('%s -- Copyright %s Nexteer',NxtrConf,first)
      | else
      |     fprintf('%s -- %s%s- %s Nexteer',NxtrConf,char(169),first,last)
      | end
  Count per uSec : Constant  Value=0.01
  Data Store Read1 : DataStoreRead  DataStoreName=SimnTi
  Data Type Conversion1 : DataTypeConversion  OutDataTypeStr=uint32
  Divide1 : Product  Inputs=**
  Divide2 : Product  Inputs=*/
  Max Counts : Constant  Value=2^32-1
  Product1 : Product
  Product2 : Product
  Rounding : Rounding
  Subtract1 : Sum  Inputs=+-
  uSec per Sec : Constant  Value=1000000
  RefTmr : Outport
  wires:
  Data Store Read1/1 -> Product1/1
  Data Type Conversion1/1 -> RefTmr/1
  uSec per Sec/1 -> Product1/2
  Count per uSec/1 -> Divide1/2
  Product1/1 -> Divide1/1
  Divide1/1 -> Subtract1/1, Divide2/1
  Max Counts/1 -> Product2/2, Divide2/2
  Divide2/1 -> Rounding/1
  Rounding/1 -> Product2/1
  Subtract1/1 -> Data Type Conversion1/1
  Product2/1 -> Subtract1/2

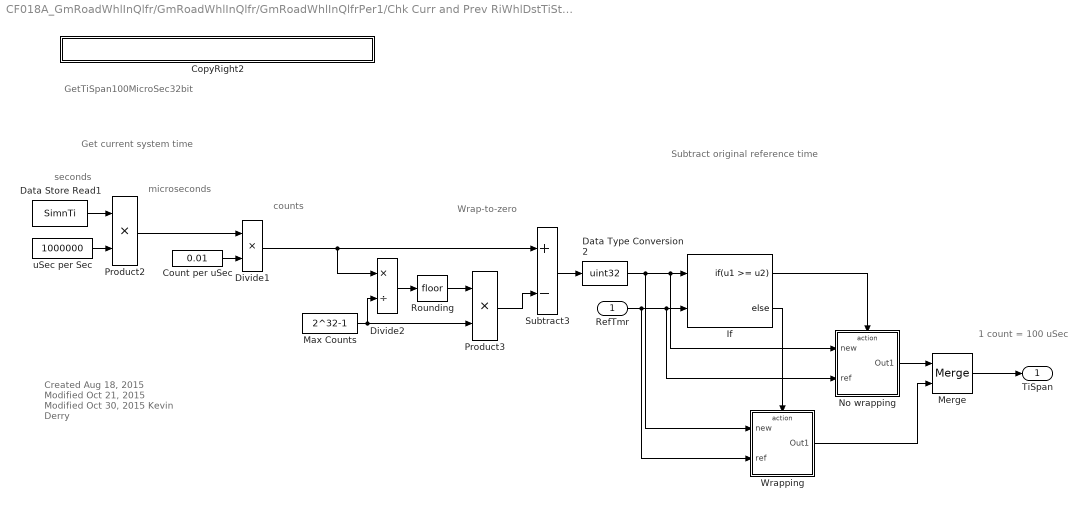
== system CF018A_GmRoadWhlInQlfr/GmRoadWhlInQlfr/GmRoadWhlInQlfrPer1/Chk Curr and Prev RiWhlDstTiStamp/Calc RiWhlFrq and RiWhlFrqVld /GetTiSpan100MicroSec32bit ==
  note: Subtract original reference time
  note: seconds
  note: microseconds
  note: counts
  note: Wrap-to-zero
  note: 1 count = 100 uSec
  note: Get current system time
  note: GetTiSpan100MicroSec32bit
  note: Created Aug 18, 2015
      | Modified Oct 21, 2015
      | Modified Oct 30, 2015
      | Kevin Derry
  RefTmr : Inport
  CopyRight2 : Subsystem  Description=|  mask(Copyright Information){none=on}
      | Copyright info block.                                               
      |                                                                     
      | Place copyright information at the top of every subsystem in design.
      mask prompts: none "No parameters"
      mask help: Place copyright information at the top of every subsystem in design.
      mask Display:
      | NxtrConf = 'Nexteer Confidential';
      | 
      | sys = bdroot; %handle for the current model ("system")
      | first = get_param(sys,'Created');
      | if(isempty(first))
      |     first = datestr(now,'yyyy');
      | else
      |     first = first(end-3:end);  %year is last four digits
      | end
      | 
      | last = get_param(sys,'LastModifiedDate');
      | if isempty(last)
      |     last = datestr(now,'yyyy');
      | else
      |     last = last(end-3:end);
      | end
      | 
      | if strcmp(first,last)
      |     fprintf('%s -- Copyright %s Nexteer',NxtrConf,first)
      | else
      |     fprintf('%s -- %s%s- %s Nexteer',NxtrConf,char(169),first,last)
      | end
  Count per uSec : Constant  Value=0.01
  Data Store Read1 : DataStoreRead  DataStoreName=SimnTi
  Data Type Conversion2 : DataTypeConversion  OutDataTypeStr=uint32
  Divide1 : Product  Inputs=**
  Divide2 : Product  Inputs=*/
  If : If  NumInputs=2  IfExpression=u1 >= u2
  Max Counts : Constant  Value=2^32-1
  Merge : Merge
  No wrapping : Subsystem  TreatAsAtomicUnit=on
  Product2 : Product
  Product3 : Product
  Rounding : Rounding
  Subtract3 : Sum  Inputs=+-
  Wrapping : Subsystem  TreatAsAtomicUnit=on
  uSec per Sec : Constant  Value=1000000
  TiSpan : Outport
  wires:
  Wrapping/1(Out1) -> Merge/2
  No wrapping/1(Out1) -> Merge/1
  If/2 -> Wrapping/Action
  If/1 -> No wrapping/Action
  Product3/1 -> Subtract3/2
  Subtract3/1 -> Data Type Conversion2/1
  Rounding/1 -> Product3/1
  Divide2/1 -> Rounding/1
  Max Counts/1 -> Divide2/2, Product3/2
  Divide1/1 -> Divide2/1, Subtract3/1
  Product2/1 -> Divide1/1
  Data Store Read1/1 -> Product2/1
  Count per uSec/1 -> Divide1/2
  uSec per Sec/1 -> Product2/2
  Merge/1 -> TiSpan/1
  RefTmr/1 -> If/2, No wrapping/2(ref), Wrapping/2(ref)
  Data Type Conversion2/1 -> If/1, No wrapping/1(new), Wrapping/1(new)

== system CF018A_GmRoadWhlInQlfr/GmRoadWhlInQlfr/GmRoadWhlInQlfrPer1/Chk Curr and Prev RiWhlDstTiStamp/Calc RiWhlFrq and RiWhlFrqVld /Prev RiWhlFrq and RiWhlFrqVld RiFrqOutOfRng to false RiFrqChgOutOfRng to false RiWhlDiagFlg to false  ==
  Action Port : ActionPort  ActionType=else
  Constant1 : Constant  Value=false  OutDataTypeStr=boolean
      settings: AttributesFormatString=%<OutDataTypeStr>
  Constant2 : Constant  Value=false  OutDataTypeStr=boolean
      settings: AttributesFormatString=%<OutDataTypeStr>
  Constant3 : Constant  Value=false  OutDataTypeStr=boolean
      settings: AttributesFormatString=%<OutDataTypeStr>
  CopyRight2 : Subsystem  Description=|  mask(Copyright Information){none=on}
      | Copyright info block.                                               
      |                                                                     
      | Place copyright information at the top of every subsystem in design.
      mask prompts: none "No parameters"
      mask help: Place copyright information at the top of every subsystem in design.
      mask Display:
      | NxtrConf = 'Nexteer Confidential';
      | 
      | sys = bdroot; %handle for the current model ("system")
      | first = get_param(sys,'Created');
      | if(isempty(first))
      |     first = datestr(now,'yyyy');
      | else
      |     first = first(end-3:end);  %year is last four digits
      | end
      | 
      | last = get_param(sys,'LastModifiedDate');
      | if isempty(last)
      |     last = datestr(now,'yyyy');
      | else
      |     last = last(end-3:end);
      | end
      | 
      | if strcmp(first,last)
      |     fprintf('%s -- Copyright %s Nexteer',NxtrConf,first)
      | else
      |     fprintf('%s -- %s%s- %s Nexteer',NxtrConf,char(169),first,last)
      | end
  Data Store Read2 : DataStoreRead  DataStoreName=PrevRiWhlFrqVld
      settings: AttributesFormatString=%<Priority>
  Data Store Read3 : DataStoreRead  DataStoreName=PrevRiWhlFrq
      settings: AttributesFormatString=%<Priority>
  RiWhlFrqVld : Outport
  RiWhlFrq : Outport  Port=2
  RiFrqOutOfRng : Outport  Port=3
  RiFrqChgOutOfRng : Outport  Port=4
  RiWhlDiagFlg : Outport  Port=5
  wires:
  Data Store Read2/1 -> RiWhlFrqVld/1
  Data Store Read3/1 -> RiWhlFrq/1
  Constant1/1 -> RiFrqOutOfRng/1
  Constant2/1 -> RiFrqChgOutOfRng/1
  Constant3/1 -> RiWhlDiagFlg/1

== system CF018A_GmRoadWhlInQlfr/GmRoadWhlInQlfr/GmRoadWhlInQlfrPer1/Chk Curr and Prev RiWhlDstTiStamp/Prev RiWhlFrq and RiWhlFrqVld RiFrqOutOfRng to false RiFrqChgOutOfRng to false RiWhlDiagFlg to false /CopyRight2 ==
